simulink model "Ex_4"  (R2019a)
settings: Solver=VariableStepAuto  StartTime=0.0  StopTime=10  RelTol=1e-3
settings Model: Creator=nth22  LastModifiedBy=nth22

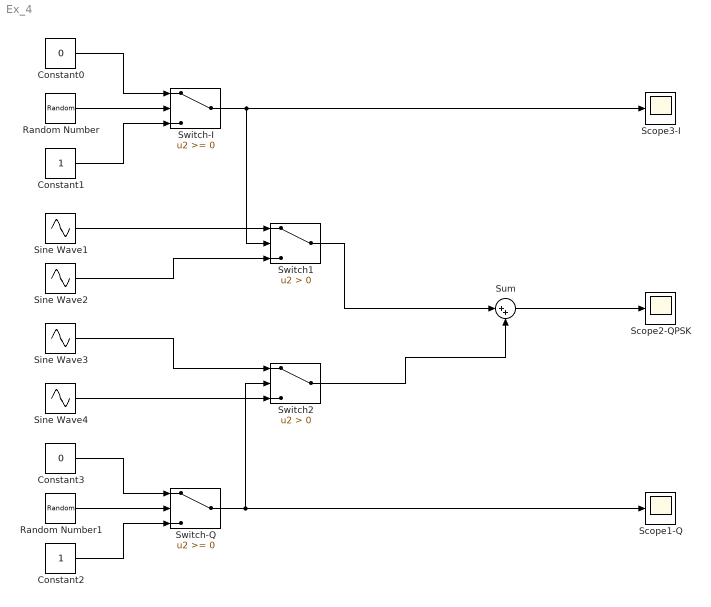
== system Ex_4 ==
  "Constant0 " : Constant  Value=0
  "Constant1 " : Constant
  "Constant2 " : Constant
  "Constant3 " : Constant  Value=0
  "Random Number " : RandomNumber  SampleTime=0.5
  "Random Number1 " : RandomNumber  SampleTime=0.5
  "Scope1-Q " : Scope
  "Scope2-QPSK " : Scope
  "Scope3-I " : Scope
  "Sine Wave1 " : Sin  Frequency=2*pi  SampleTime=0.001
  "Sine Wave2 " : Sin  Frequency=2*pi  Phase=3*pi/2  SampleTime=0.001
  "Sine Wave3 " : Sin  Frequency=2*pi  Phase=pi/2  SampleTime=0.001
  "Sine Wave4 " : Sin  Frequency=2*pi  Phase=pi  SampleTime=0.001  VectorParams1D=off
  Sum : Sum  Inputs=|++
  "Switch-I " : Switch
  Switch-Q : Switch
  "Switch1 " : Switch  Criteria=u2 > Threshold
  "Switch2 " : Switch  Criteria=u2 > Threshold
  wires:
  "Constant3 "/1 -> Switch-Q/1
  "Random Number1 "/1 -> Switch-Q/2
  "Constant2 "/1 -> Switch-Q/3
  "Constant1 "/1 -> "Switch-I "/3
  "Constant0 "/1 -> "Switch-I "/1
  "Random Number "/1 -> "Switch-I "/2
  "Switch-I "/1 -> "Scope3-I "/1, "Switch1 "/2
  Switch-Q/1 -> "Switch2 "/2, "Scope1-Q "/1
  "Sine Wave3 "/1 -> "Switch2 "/1
  "Sine Wave4 "/1 -> "Switch2 "/3
  "Sine Wave2 "/1 -> "Switch1 "/3
  "Sine Wave1 "/1 -> "Switch1 "/1
  Sum/1 -> "Scope2-QPSK "/1
  "Switch2 "/1 -> Sum/2
  "Switch1 "/1 -> Sum/1
